simulink model "bic"  (R2018a)
settings: Solver=FixedStepAuto  StartTime=0.0  StopTime=10.0  FixedStep=Ts  RelTol=1e-3  EnableMultiTasking=on
values from neighbouring files (symbols this model uses):
  delta_f = alpha    [sim_veh_MPC.m]    (also in sim_veh_MPC_smooth.m = gain*smooth_steering([delta_h,alpha]))
  psi0 = psi    (= 0)    [sim_veh_MPC.m]    (also in sim_veh_MPC_smooth.m)
  v0 = memory(4)    [controller.m]    (also in controller_lqr.m = memory(5); controller_lqr2.m = v; controller_mpc_Tunner.m = v)
  x_car0 = x_car    (= 0)    [sim_veh_MPC.m]    (also in sim_veh_MPC_smooth.m)
  y_car0 = y_car    (= 0)    [sim_veh_MPC.m]    (also in sim_veh_MPC_smooth.m)
undefined symbols (not defined in the file or in its folder): acc
libraries: simulink x1
settings Model: Creator=Administrator  LastModifiedBy=berlin
settings DataIOCC: LimitDataPoints=on  SaveFormat=Array
settings OptimizationCC: LifeSpan=inf
settings DebuggingCC: SolverPrmCheckMsg=warning  SFUnexpectedBacktrackingDiag=warning  SFNoUnconditionalDefaultTransitionDiag=warning  SFExecutionAtInitializationDiag=none
settings HardwareCC: ProdBitPerPointer=32  ProdBitPerSizeT=32  ProdBitPerPtrDiffT=32  ProdLargestAtomicFloat=None  ProdIntDivRoundTo=Undefined  ProdEndianess=Unspecified  ProdWordSize=32  ProdHWDeviceType=32-bit Generic
settings ModelReferenceCC: PropagateSignalLabelsOutOfModel=off
settings CodeAppCC: StateflowObjectComments=on
settings GRTTargetCC: TargetLangStandard=C89/C90 (ANSI)  GeneratePreprocessorConditionals=Disable all
settings ConfigComp: CovMetricSettings=dw  CovHtmlReporting=on  CovSaveCumulativeToWorkspaceVar=on  CovSaveSingleToWorkspaceVar=on  CovExternalEMLEnable=off  CovSFcnEnable=off

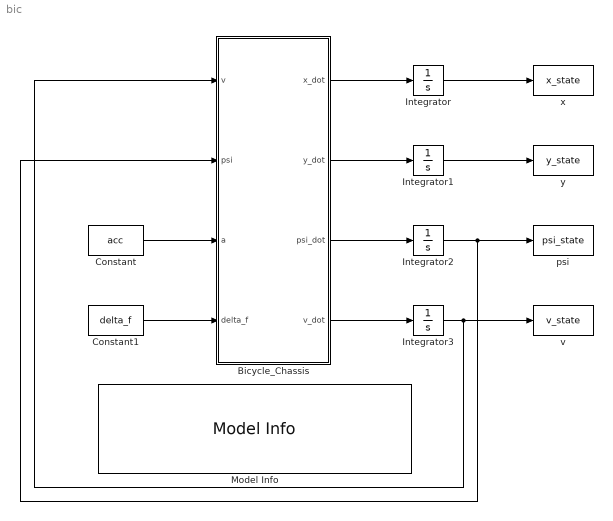
== system bic ==
  " Bicycle_Chassis" : MATLAB Function  TreatAsAtomicUnit=on
  Constant : Constant  Value=acc
  Constant1 : Constant  Value=delta_f
  Integrator : Integrator  InitialCondition=x_car0
  Integrator1 : Integrator  InitialCondition=y_car0
  Integrator2 : Integrator  InitialCondition=psi0
  Integrator3 : Integrator  InitialCondition=v0
  Model Info : simulink/Model-Wide Utilities/Model Info  Frame=on  DisplayStringWithTags=|  HorizontalTextAlignment=Left  LeftAlignmentValue=0.02
      | Model Info
      | 
      | [delta_f] is the steering angle on the front wheels.
      | Closewise is Positive.
      | 
      | [acc] is the acceleration requirement.
  psi : ToWorkspace  VariableName=psi_state  SaveFormat=Timeseries  SampleTime=-1
  v : ToWorkspace  VariableName=v_state  SaveFormat=Timeseries  SampleTime=-1
  x : ToWorkspace  VariableName=x_state  SaveFormat=Timeseries  SampleTime=-1
  y : ToWorkspace  VariableName=y_state  SaveFormat=Timeseries  SampleTime=-1
  wires:
  " Bicycle_Chassis"/1(x_dot) -> Integrator/1
  " Bicycle_Chassis"/2(y_dot) -> Integrator1/1
  " Bicycle_Chassis"/3(psi_dot) -> Integrator2/1
  " Bicycle_Chassis"/4(v_dot) -> Integrator3/1
  Integrator3/1 -> v/1, " Bicycle_Chassis"/1(v)
  Integrator2/1 -> psi/1, " Bicycle_Chassis"/2(psi)
  Integrator/1 -> x/1
  Integrator1/1 -> y/1
  Constant/1 -> " Bicycle_Chassis"/3(a)
  Constant1/1 -> " Bicycle_Chassis"/4(delta_f)

== matlab function bic/ Bicycle_Chassis ==
  data: v input; x_dot output; psi input; a input; delta_f input; y_dot output; psi_dot output; v_dot output
function [x_dot,y_dot,psi_dot,v_dot] = bicycle(v, psi,a,delta_f)

lr = 1.6;
lf = 1.4;
wb = lr+lf;
beta = atan(lr/wb*tan(delta_f));

x_dot = v*cos(psi+ beta);
y_dot = v*sin(psi+beta);
psi_dot= v/lr*sin(beta);
v_dot = a;

end

%% ref: http://www.me.berkeley.edu/~frborrel/pdfpub/IV_KinematicMPC_jason.pdf
